simulink model "poczatkoweodpalenie"  (R2015a)
settings: Solver=ode3  StartTime=0.0  StopTime=600  FixedStep=0.01  RelTol=1e-3
undefined symbols (not defined in the file or in its folder): a, a1, a2, a3, b, c, C1, C2, C3, h2max, q, R, w
libraries: simulink x1
settings Model: Creator=Student  LastModifiedBy=Student

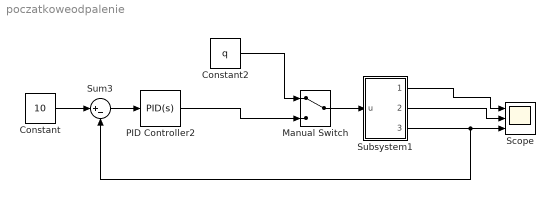
== system poczatkoweodpalenie ==
  Constant : Constant  Value=10
  Constant2 : Constant  Value=q
  Manual Switch : ManualSwitch
  PID Controller2 : simulink/Continuous/PID Controller  Controller=PID  TimeDomain=Continuous-time  SampleTime=-1  IntegratorMethod=Forward Euler  FilterMethod=Forward Euler  Form=Parallel  UseFilter=on  ControllerParametersSource=internal  P=6253.07553913147  I=38.0638936363756  D=255497.726155373  N=2.40668732962837  InitialConditionSource=internal  InitialConditionForIntegrator=0  InitialConditionForFilter=0  ExternalReset=none  LimitOutput=on  UpperSaturationLimit=160  LowerSaturationLimit=0  LinearizeAsGain=on  AntiWindupMode=none  Kb=1  TrackingMode=off  Kt=1  PParamMin=[]  PParamMax=[]  IParamMin=[]  IParamMax=[]  DParamMin=[]  DParamMax=[]  NParamMin=[]  NParamMax=[]  KbParamMin=[]  KbParamMax=[]  KtParamMin=[]  KtParamMax=[]  POutMin=[]  POutMax=[]  IOutMin=[]  IOutMax=[]  DOutMin=[]  DOutMax=[]  NOutMin=[]  NOutMax=[]  KbOutMin=[]  KbOutMax=[]  KtOutMin=[]  KtOutMax=[]  IntegratorOutMin=[]  IntegratorOutMax=[]  FilterOutMin=[]  FilterOutMax=[]  SumOutMin=[]  SumOutMax=[]  SumI1OutMin=[]  SumI1OutMax=[]  SumI2OutMin=[]  SumI2OutMax=[]  SumI3OutMin=[]  SumI3OutMax=[]  SumDOutMin=[]  SumDOutMax=[]  SaturationOutMin=[]  SaturationOutMax=[]  IntegratorContinuousStateAttributes=''  IntegratorStateMustResolveToSignalObject=off  IntegratorRTWStateStorageClass=Auto  FilterContinuousStateAttributes=''  FilterStateMustResolveToSignalObject=off  FilterRTWStateStorageClass=Auto  DifferentiatorICPrevScaledInput=0  DifferentiatorOutMin=[]  DifferentiatorOutMax=[]
  Scope : Scope  NumInputPorts=3
      settings: YMin=-5~-5~-5  YMax=5~5~5  SaveName=zbiorniki
  Subsystem1 : Subsystem
  Sum3 : Sum  Inputs=|+-
  wires:
  Subsystem1/1(h1out) -> Scope/1
  Subsystem1/2("h2out ") -> Scope/2
  Subsystem1/3("h3out ") -> Sum3/2, Scope/3
  Constant/1 -> Sum3/1
  Sum3/1 -> PID Controller2/1
  PID Controller2/1 -> Manual Switch/2
  Manual Switch/1 -> Subsystem1/1(u)
  Constant2/1 -> Manual Switch/1

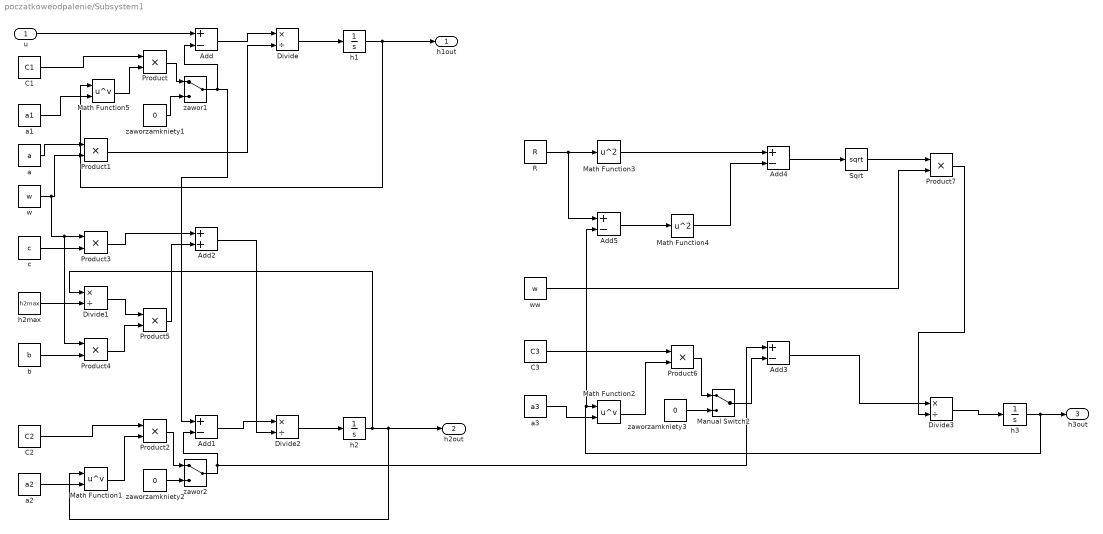
== system poczatkoweodpalenie/Subsystem1 ==
  u : Inport
  Add{,1,3..5} (5 alike) : Sum  Inputs=+-
  Add2 : Sum
  C1 : Constant  Value=C1
  C2 : Constant  Value=C2
  C3 : Constant  Value=C3
  Divide{,1..3} (4 alike) : Product  Inputs=*/
  Manual Switch2 : ManualSwitch
  Math Function1 : Math  Operator=pow  SaturateOnIntegerOverflow=on
  Math Function2 : Math  Operator=pow  SaturateOnIntegerOverflow=on
  Math Function3 : Math  Operator=square  SaturateOnIntegerOverflow=on
  Math Function4 : Math  Operator=square  SaturateOnIntegerOverflow=on
  Math Function5 : Math  Operator=pow  SaturateOnIntegerOverflow=on
  Product{,1..7} (8 alike) : Product
  R : Constant  Value=R
  Sqrt : Sqrt  SaturateOnIntegerOverflow=on
  a : Constant  Value=a
  a1 : Constant  Value=a1
  a2 : Constant  Value=a2
  a3 : Constant  Value=a3
  b : Constant  Value=b
  c : Constant  Value=c
  h1 : Integrator  LimitOutput=on  UpperSaturationLimit=35  LowerSaturationLimit=0
  h2 : Integrator  LimitOutput=on  UpperSaturationLimit=35  LowerSaturationLimit=0
  h2max : Constant  Value=h2max
  h3 : Integrator  InitialCondition=2  LimitOutput=on  UpperSaturationLimit=35  LowerSaturationLimit=0
  w : Constant  Value=w
  ww : Constant  Value=w
  "zawor1 " : ManualSwitch
  "zawor2 " : ManualSwitch
  zaworzamkniety1 : Constant  Value=0
  zaworzamkniety2 : Constant  Value=0
  zaworzamkniety3 : Constant  Value=0
  h1out : Outport
  "h2out " : Outport  Port=2
  "h3out " : Outport  Port=3
  wires:
  h1/1 -> Math Function5/1, h1out/1
  h2/1 -> Divide1/1, "h2out "/1, Math Function1/1
  Math Function1/1 -> Product2/2
  u/1 -> Add/1
  Add/1 -> Divide/1
  Product/1 -> "zawor1 "/1
  C1/1 -> Product/1
  a/1 -> Product1/1
  Product4/1 -> Product5/2
  Product1/1 -> Divide/2
  h2max/1 -> Divide1/2
  C2/1 -> Product2/1
  w/1 -> Product4/1, Product3/1, Product1/2
  Divide2/1 -> h2/1
  Product7/1 -> Divide3/2
  Add2/1 -> Divide2/2
  Divide1/1 -> Product5/1
  a2/1 -> Math Function1/2
  Product5/1 -> Add2/2
  Add3/1 -> Divide3/1
  R/1 -> Add5/1, Math Function3/1
  h3/1 -> "h3out "/1, Add5/2, Math Function2/1
  Math Function3/1 -> Add4/1
  Add4/1 -> Sqrt/1
  Divide3/1 -> h3/1
  Sqrt/1 -> Product7/1
  Math Function2/1 -> Product6/2
  b/1 -> Product4/2
  Add5/1 -> Math Function4/1
  a3/1 -> Math Function2/2
  Product3/1 -> Add2/1
  C3/1 -> Product6/1
  ww/1 -> Product7/2
  Math Function4/1 -> Add4/2
  Add1/1 -> Divide2/1
  c/1 -> Product3/2
  zaworzamkniety1/1 -> "zawor1 "/2
  "zawor1 "/1 -> Add1/1, Add/2
  Product2/1 -> "zawor2 "/1
  zaworzamkniety2/1 -> "zawor2 "/2
  "zawor2 "/1 -> Add3/1, Add1/2
  Product6/1 -> Manual Switch2/1
  zaworzamkniety3/1 -> Manual Switch2/2
  Manual Switch2/1 -> Add3/2
  Divide/1 -> h1/1
  a1/1 -> Math Function5/2
  Math Function5/1 -> Product/2
